simulink model "TADPOLE_Closed_Loop"  (R2024b)
settings: Solver=FixedStepAuto  StartTime=0.0  StopTime=19  RelTol=1e-3
InitFcn:
  | clear mex;
values from neighbouring files (symbols this model uses):
  timeDelta = 1/500    (= 0.002)    [TADPOLEControl.m]
settings Model: Creator=pplat  LastModifiedBy=pplat
settings DebuggingCC: AlgebraicLoopMsg=none

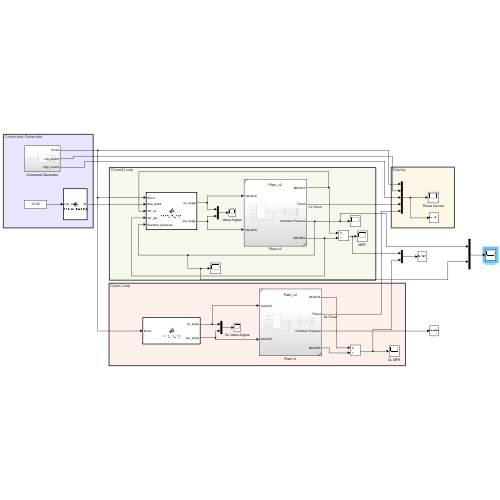
[thumbnail: Simulink's stored preview of the top-level diagram]
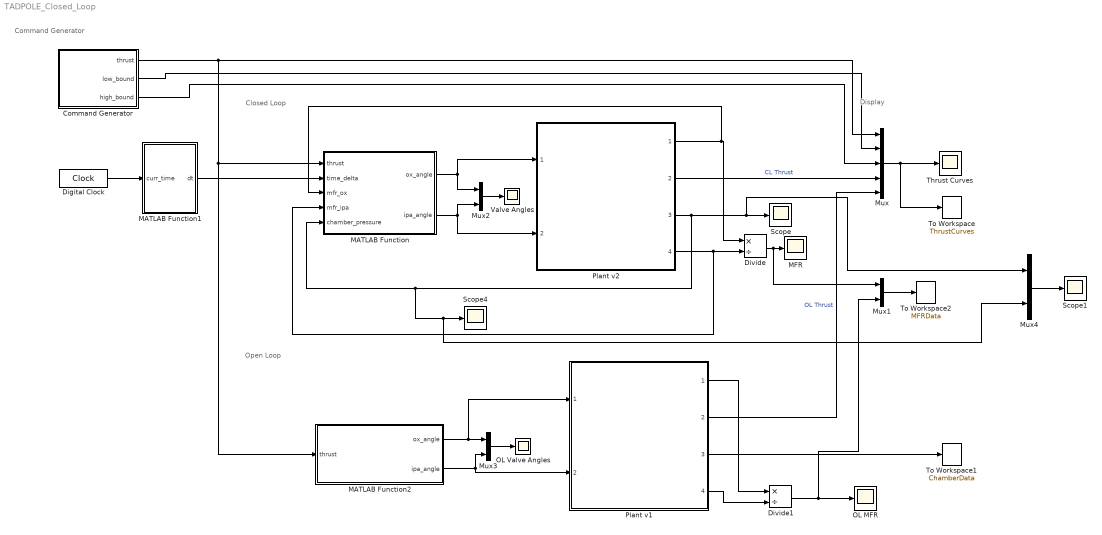
== system TADPOLE_Closed_Loop ==
  note: Display
  note: Open Loop
  note: Closed Loop
  note: Command Generator
  Command Generator : Subsystem
  Digital Clock : DigitalClock  SampleTime=timeDelta
  Divide : Product  Inputs=*/
  Divide1 : Product  Inputs=*/
  MATLAB Function : MATLAB Function  TreatAsAtomicUnit=on
  MATLAB Function1 : MATLAB Function  TreatAsAtomicUnit=on
  MATLAB Function2 : MATLAB Function  TreatAsAtomicUnit=on
  MFR : Scope
  Mux : Mux  Inputs=5
  Mux{1..4} (4 alike) : Mux  Inputs=2
  OL MFR : Scope
  OL Valve Angles : Scope
  Plant v1 : Subsystem  ReferencedSubsystem=Plant_v2
  Plant v2 : Subsystem  ReferencedSubsystem=Plant_v2
  Scope : Scope
  Scope1 : Scope
  Scope4 : Scope
  Thrust Curves : Scope
  To Workspace : ToWorkspace  VariableName=ThrustCurves  SaveFormat=Timeseries  SampleTime=-1
  To Workspace1 : ToWorkspace  VariableName=ChamberData  SaveFormat=Timeseries  SampleTime=-1
  To Workspace2 : ToWorkspace  VariableName=MFRData  SaveFormat=Timeseries  SampleTime=-1
  Valve Angles : Scope
  wires:
  Mux/1 -> To Workspace/1, Thrust Curves/1
  Plant v2/1 -> MATLAB Function/3(mfr_ox), Divide/1
  Plant v2/4 -> MATLAB Function/4(mfr_ipa), Divide/2
  MATLAB Function/2(ipa_angle) -> Plant v2/2, Mux2/2
  MATLAB Function/1(ox_angle) -> Plant v2/1, Mux2/1
  Mux2/1 -> Valve Angles/1
  Divide/1 -> Mux1/1, MFR/1
  Command Generator/1(thrust) -> Mux/1, MATLAB Function2/1(thrust), MATLAB Function/1(thrust)
  Plant v2/2 -> Mux/4  "CL Thrust"
  Command Generator/2(low_bound) -> Mux/2
  Command Generator/3(high_bound) -> Mux/3
  MATLAB Function1/1(dt) -> MATLAB Function/2(time_delta)
  Mux3/1 -> OL Valve Angles/1
  Divide1/1 -> Mux1/2, OL MFR/1
  MATLAB Function2/1(ox_angle) -> Mux3/1, Plant v1/1
  MATLAB Function2/2(ipa_angle) -> Plant v1/2, Mux3/2
  Digital Clock/1 -> MATLAB Function1/1(curr_time)
  Plant v1/1 -> Divide1/1
  Plant v1/4 -> Divide1/2
  Plant v1/2 -> Mux/5  "OL Thrust"
  Mux1/1 -> To Workspace2/1
  Plant v2/3 -> Mux4/2, Scope4/1, MATLAB Function/5(chamber_pressure), Mux4/1, Scope/1
  Mux4/1 -> Scope1/1
  Plant v1/3 -> To Workspace1/1

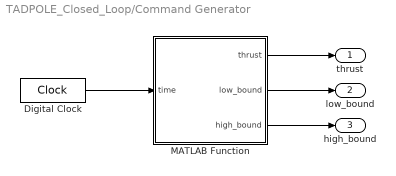
== system TADPOLE_Closed_Loop/Command Generator ==
  Digital Clock : DigitalClock  SampleTime=timeDelta
  MATLAB Function : MATLAB Function  TreatAsAtomicUnit=on
  thrust : Outport
  low_bound : Outport  Port=2
  high_bound : Outport  Port=3
  wires:
  MATLAB Function/1(thrust) -> thrust/1
  Digital Clock/1 -> MATLAB Function/1(time)
  MATLAB Function/2(low_bound) -> low_bound/1
  MATLAB Function/3(high_bound) -> high_bound/1

== matlab function TADPOLE_Closed_Loop/MATLAB Function ==
  data: thrust input; time_delta input; ox_angle output; ipa_angle output; mfr_ox input; mfr_ipa input; chamber_pressure input
function [ox_angle, ipa_angle] = send_to_cpp(thrust, time_delta, mfr_ox, mfr_ipa, chamber_pressure)
coder.extrinsic('closed_loop_valve_control_wrap');  % Declare MEX function as extrinsic
ox_angle = 0;
ipa_angle = 0;
[ox_angle, ipa_angle] = closed_loop_valve_control_wrap(thrust, time_delta, mfr_ox, mfr_ipa, chamber_pressure);

== matlab function TADPOLE_Closed_Loop/MATLAB Function1 ==
  data: dt output; curr_time input
function dt = measure_timestep(curr_time)
    persistent prev_time;
    if isempty(prev_time)
        prev_time = 0;
    end
    if curr_time < 0.3
        dt = 0;
    else
        dt = curr_time - prev_time;
    end
    prev_time = curr_time;
end

== matlab function TADPOLE_Closed_Loop/Command Generator/MATLAB Function ==
  data: time input; thrust output; low_bound output; high_bound output
function [thrust,low_bound,high_bound] = thrustCurveBounds(time)
thrust = test3(time);
t_past = test3(time - 0.5);
t_future = test3(time + 0.5);

high_bound = max([thrust, t_past, t_future]) + 0.05 * 550;
low_bound = min([thrust, t_past, t_future]) - 0.05 * 550;

end

== matlab function TADPOLE_Closed_Loop/MATLAB Function2 ==
  data: thrust input; ox_angle output; ipa_angle output
function [ox_angle, ipa_angle] = send_to_cpp(thrust)
coder.extrinsic('open_loop_valve_control_wrap');  % Declare MEX function as extrinsic
ox_angle = 0;
ipa_angle = 0;
[ox_angle, ipa_angle] = open_loop_valve_control_wrap(thrust);
